simulink model "Hil_Climbers_Integrated_V5"  (R2021a)
settings: Solver=VariableStepAuto  StartTime=0.0  StopTime=10.0  RelTol=1e-3
settings Model: Creator=Sai229  LastModifiedBy=achu

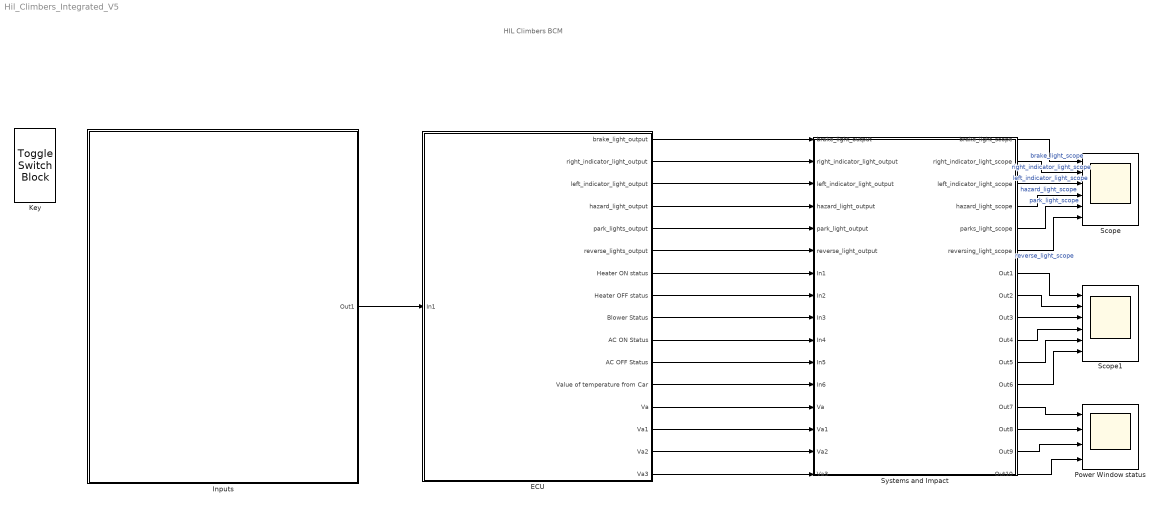
== system Hil_Climbers_Integrated_V5 ==
  note: HIL Climbers BCM
  " ECU" : Subsystem
  Inputs : Subsystem
  Key : ToggleSwitchBlock  LabelPosition=Hide
      settings: Values={{'Off', 'On'}, [0 1]}
  Power Window status : Scope  NumInputPorts=4
  Scope : Scope  NumInputPorts=6
  Scope1 : Scope  NumInputPorts=6
  Systems and Impact : Subsystem
  wires:
  Systems and Impact/12(Out6) -> Scope1/6
  Systems and Impact/11(Out5) -> Scope1/5
  Systems and Impact/10(Out4) -> Scope1/4
  Systems and Impact/1(brake_light_scope) -> Scope/1  "brake_light_scope"
  Systems and Impact/9(Out3) -> Scope1/3
  Systems and Impact/8(Out2) -> Scope1/2
  Systems and Impact/5(parks_light_scope) -> Scope/5  "park_light_scope"
  Systems and Impact/7(Out1) -> Scope1/1
  Systems and Impact/4(hazard_light_scope) -> Scope/4  "hazard_light_scope"
  Systems and Impact/6(reversing_light_scope) -> Scope/6  "reverse_light_scope"
  Systems and Impact/3(left_indicator_light_scope) -> Scope/3  "left_indicator_light_scope"
  Systems and Impact/2(right_indicator_light_scope) -> Scope/2  "right_indicator_light_scope"
  " ECU"/1(brake_light_output) -> Systems and Impact/1(brake_light_output)
  " ECU"/2(right_indicator_light_output) -> Systems and Impact/2(right_indicator_light_output)
  " ECU"/3(left_indicator_light_output) -> Systems and Impact/3(left_indicator_light_output)
  " ECU"/4(hazard_light_output) -> Systems and Impact/4(hazard_light_output)
  " ECU"/5(park_lights_output) -> Systems and Impact/5(park_light_output)
  " ECU"/6(reverse_lights_output) -> Systems and Impact/6(reverse_light_output)
  " ECU"/7(Heater ON status) -> Systems and Impact/7(In1)
  " ECU"/8(Heater OFF status) -> Systems and Impact/8(In2)
  " ECU"/9(Blower Status) -> Systems and Impact/9(In3)
  " ECU"/10(AC ON Status) -> Systems and Impact/10(In4)
  " ECU"/11(AC OFF Status) -> Systems and Impact/11(In5)
  " ECU"/12(Value of temperature from Car) -> Systems and Impact/12(In6)
  " ECU"/13(Va) -> Systems and Impact/13(Va)
  " ECU"/14(Va1) -> Systems and Impact/14(Va1)
  " ECU"/15(Va2) -> Systems and Impact/15(Va2)
  " ECU"/16(Va3) -> Systems and Impact/16(Va3)
  Systems and Impact/13(Out7) -> Power Window status/1
  Systems and Impact/14(Out8) -> Power Window status/2
  Systems and Impact/15(Out9) -> Power Window status/3
  Systems and Impact/16(Out10) -> Power Window status/4
  Inputs/1(Out1) -> " ECU"/1(In1)

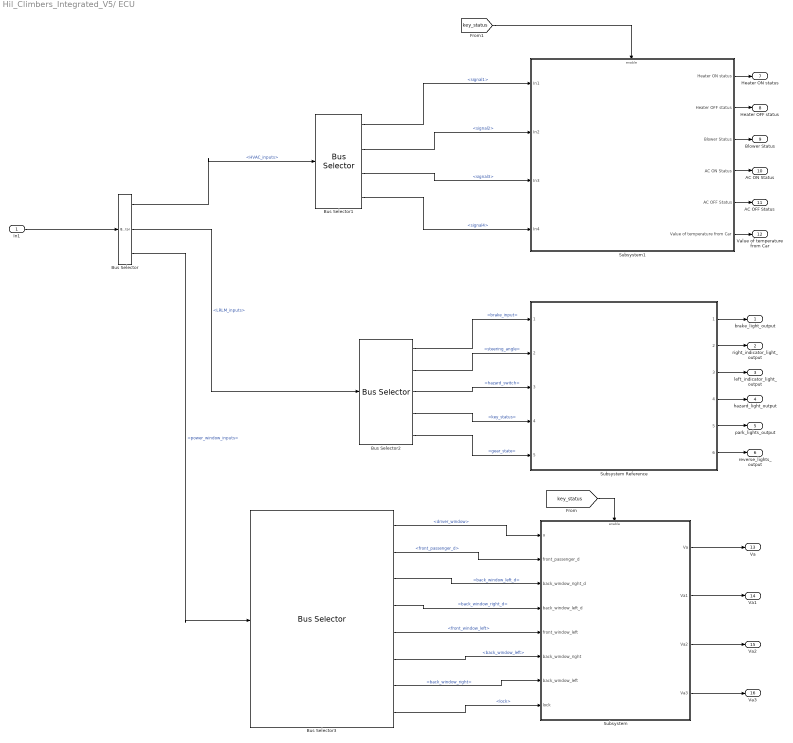
== system Hil_Climbers_Integrated_V5/ ECU ==
  In1 : Inport
  Bus Selector : BusSelector  OutputSignals=HVAC_inputs,LRLM_inputs,power_window_inputs
  Bus Selector1 : BusSelector  OutputSignals=signal1,signal2,signal3,signal4
  Bus Selector2 : BusSelector  OutputSignals=brake_input,steering_angle,hazard_switch,key_status,gear_state
  Bus Selector3 : BusSelector  OutputSignals=driver_window,front_passenger_d,back_window_left_d,back_window_right_d,front_window_left,back_window_left,back_window_right,lock
  Subsystem : Subsystem
  Subsystem Reference : Subsystem  ReferencedSubsystem=LRLM_ECU
  Subsystem1 : Subsystem
  brake_light_output : Outport
  right_indicator_light_output : Outport  Port=2
  left_indicator_light_output : Outport  Port=3
  hazard_light_output : Outport  Port=4
  park_lights_output : Outport  Port=5
  reverse_lights_output : Outport  Port=6
  Heater ON status : Outport  Port=7
  Heater OFF status : Outport  Port=8
  Blower Status : Outport  Port=9
  AC ON Status : Outport  Port=10
  AC OFF Status : Outport  Port=11
  Value of temperature from Car : Outport  Port=12
  Va : Outport  Port=13
  Va1 : Outport  Port=14
  Va2 : Outport  Port=15
  Va3 : Outport  Port=16
  wires:
  Subsystem Reference/5 -> park_lights_output/1
  Subsystem Reference/3 -> left_indicator_light_output/1
  Subsystem Reference/6 -> reverse_lights_output/1
  Subsystem Reference/1 -> brake_light_output/1
  Subsystem Reference/2 -> right_indicator_light_output/1
  Subsystem Reference/4 -> hazard_light_output/1
  Subsystem/1(Va) -> Va/1
  Subsystem/2(Va1) -> Va1/1
  Subsystem/3(Va2) -> Va2/1
  Subsystem/4(Va3) -> Va3/1
  Subsystem1/1(Heater ON status) -> Heater ON status/1
  Subsystem1/2(Heater OFF status) -> Heater OFF status/1
  Subsystem1/3(Blower Status) -> Blower Status/1
  Subsystem1/4(AC ON Status) -> AC ON Status/1
  Subsystem1/5(AC OFF Status) -> AC OFF Status/1
  Subsystem1/6(Value of temperature from Car) -> Value of temperature from Car/1
  [key_status] -> Subsystem1/Enable
  In1/1 -> Bus Selector/1
  Bus Selector/1 -> Bus Selector1/1  "<HVAC_inputs>"
  Bus Selector/2 -> Bus Selector2/1  "<LRLM_inputs>"
  Bus Selector/3 -> Bus Selector3/1  "<power_window_inputs>"
  Bus Selector1/1 -> Subsystem1/1(In1)  "<signal1>"
  Bus Selector1/2 -> Subsystem1/2(In2)  "<signal2>"
  Bus Selector1/3 -> Subsystem1/3(In3)  "<signal3>"
  Bus Selector1/4 -> Subsystem1/4(In4)  "<signal4>"
  Bus Selector3/1 -> Subsystem/1(u)  "<driver_window>"
  Bus Selector3/2 -> Subsystem/2(front_passenger_d)  "<front_passenger_d>"
  Bus Selector3/3 -> Subsystem/3(back_window_right_d)  "<back_window_left_d>"
  Bus Selector3/4 -> Subsystem/4(back_window_left_d)  "<back_window_right_d>"
  Bus Selector3/5 -> Subsystem/5(front_window_left)  "<front_window_left>"
  Bus Selector3/6 -> Subsystem/6(back_window_right)  "<back_window_left>"
  Bus Selector3/7 -> Subsystem/7(back_window_left)  "<back_window_right>"
  Bus Selector3/8 -> Subsystem/8(lock)  "<lock>"
  Bus Selector2/1 -> Subsystem Reference/1  "<brake_input>"
  Bus Selector2/2 -> Subsystem Reference/2  "<steering_angle>"
  Bus Selector2/3 -> Subsystem Reference/3  "<hazard_switch>"
  Bus Selector2/4 -> Subsystem Reference/4  "<key_status>"
  Bus Selector2/5 -> Subsystem Reference/5  "<gear_state>"
  [key_status] -> Subsystem/Enable

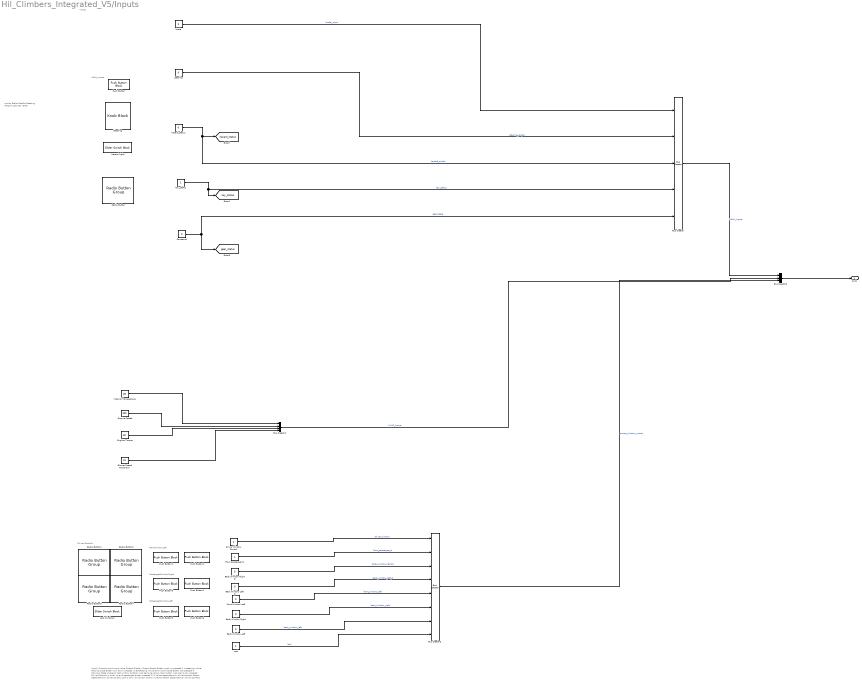
== system Hil_Climbers_Integrated_V5/Inputs ==
  note: Inputs
  note: LRLM_inputs
  note: Inputs:
      | Brake Paddle
      | Steering
      | Hazard Light
      | Key
      | Gear
  note: PsssengertWindowLeft
  note: FrontWindowLeft
  note: Driver Controls
  note: Input / Outputs
      |
      | Input
      | Input value
      | Output Display
      | Output Graph
      |
      | Button push up pressed
      | 1
      | Increasing value
      | Raising slope
      |
      | Button pull down pressed
      | -1
      | Decreasing value
      | Downward slope
      |
      | Button not pressed
      | 0
      | Previous state wherever last window position was
      | Same level as when button was previously pressed
      |
      | Driver Controls in push up and passenger button pressed
      | 1/-1
      | Value dependent on driver controls
      | Graph dependent on driver controls
      |
      | Lock
      | 1
      | Only driver can control windows
      | Graph dependent on driver controls
  note: PsssengertWindowRight
  Back Window Left : Constant  Value=0
  Back Window Left D : Constant  Value=0
  Back Window Right : Constant  Value=0
  Back Window Right D : Constant  Value=0
  Blower Speed Proportion : Constant  Value=10
  Bus Creator : BusCreator  Inputs=5
  Bus Creator1 : BusCreator  Inputs=4
  Bus Creator2 : BusCreator  Inputs=8
  Bus Creator3 : BusCreator  Inputs=3
  Constant4 : Constant  Value=0
  Driver Window Control : Constant
  Engine Speed : Constant  Value=100
  Engine Torque : Constant  Value=30
  Front Window Left : Constant  Value=0
  Front passenger D : Constant
  Hazard Light : SliderSwitchBlock  LabelPosition=Hide
      settings: Values={{'Off', 'On'}, [0 1]}
  Internal Temperature : Constant  Value=28
  Lock : Constant
  Lock Windows : SliderSwitchBlock
      settings: Values={{'Unlock', 'Lock'}, [0 1]}
  Push Button : PushButtonBlock  ButtonText=Brake
  Push Button1 : PushButtonBlock  ButtonText=Push up window
  Push Button2 : PushButtonBlock  ButtonText=Pull down window  OnValue=-1
  Push Button3 : PushButtonBlock  ButtonText=Push up window
  Push Button4 : PushButtonBlock  ButtonText=Pull down window  OnValue=-1
  Push Button5 : PushButtonBlock  ButtonText=Push up window
  Push Button6 : PushButtonBlock  ButtonText=Pull down window  OnValue=-1
  Radio Button : RadioButtonGroup  LabelPosition=Hide  SelectedLabel=Neutral  ButtonGroupName=Gear
      settings: Values={{'Neutral', 'Drive', 'Park', 'Reverse'}, [0 1 2 3]}
  Radio Button1 : RadioButtonGroup  LabelPosition=Hide  SelectedLabel=Open  ButtonGroupName=Driver Window Controls
      settings: Values={{'Open', 'Stop', 'Close'}, [1 0 -1]}
  Radio Button2 : RadioButtonGroup  LabelPosition=Hide  SelectedLabel=Open  ButtonGroupName=Front Passenger
      settings: Values={{'Open', 'Stop', 'Close'}, [1 0 -1]}
  Radio Button3 : RadioButtonGroup  LabelPosition=Hide  SelectedLabel=Stop  ButtonGroupName=Back Window Right
      settings: Values={{'Open', 'Stop', 'Close'}, [1 0 -1]}
  Radio Button4 : RadioButtonGroup  LabelPosition=Hide  SelectedLabel=Stop  ButtonGroupName=Back Window Left
      settings: Values={{'Open', 'Stop', 'Close'}, [1 0 -1]}
  Steering : KnobBlock  LabelPosition=Hide  ScaleMin=-50  ScaleMax=50  TickInterval=10
  brake : Constant  Value=0
  hazard_status : Constant  Value=0
  key_status : Constant
  steering : Constant  Value=0
  Out1 : Outport
  tag scope: gear_status=global, hazard_status=global, key_status=global
  wires:
  brake/1 -> Bus Creator/1  "brake_input"
  Constant4/1 -> Bus Creator/5, [gear_status]  "gear_state"
  steering/1 -> Bus Creator/2  "steering_angle"
  key_status/1 -> Bus Creator/4, [key_status]  "key_status"
  hazard_status/1 -> [hazard_status], Bus Creator/3  "hazard_switch"
  Internal Temperature/1 -> Bus Creator1/1
  Engine Speed/1 -> Bus Creator1/2
  Engine Torque/1 -> Bus Creator1/3
  Blower Speed Proportion/1 -> Bus Creator1/4
  Driver Window Control/1 -> Bus Creator2/1  "driver_window"
  Front passenger D/1 -> Bus Creator2/2  "front_passenger_d"
  Back Window Right D/1 -> Bus Creator2/3  "back_window_right_d"
  Back Window Left D/1 -> Bus Creator2/4  "back_window_left_d"
  Front Window Left/1 -> Bus Creator2/5  "front_window_left"
  Back Window Right/1 -> Bus Creator2/6  "back_window_right"
  Back Window Left/1 -> Bus Creator2/7  "back_window_left"
  Lock/1 -> Bus Creator2/8  "lock"
  Bus Creator/1 -> Bus Creator3/1  "LRLM_inputs"
  Bus Creator1/1 -> Bus Creator3/2  "HVAC_inputs"
  Bus Creator2/1 -> Bus Creator3/3  "power_window_inputs"
  Bus Creator3/1 -> Out1/1

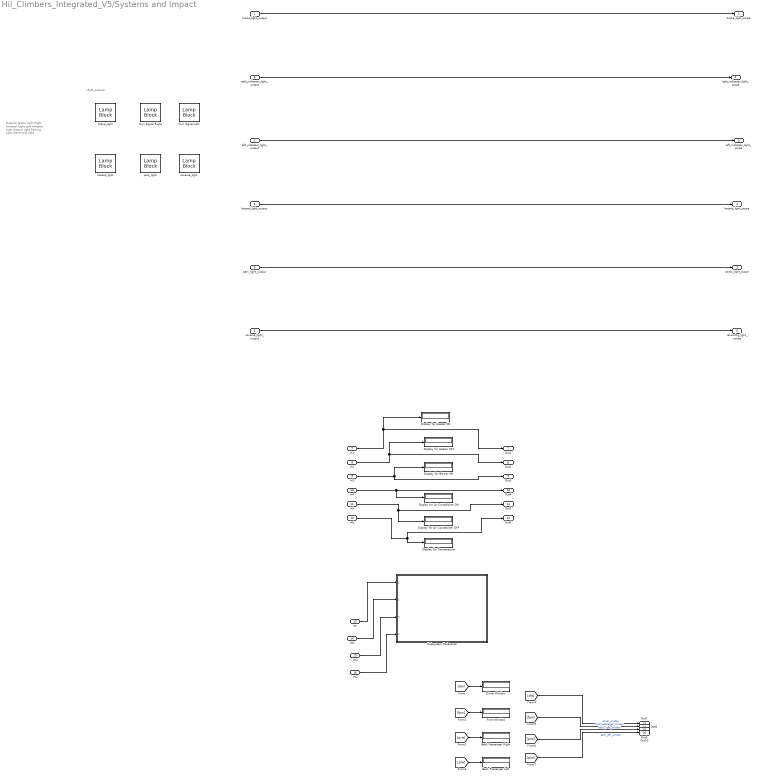
== system Hil_Climbers_Integrated_V5/Systems and Impact ==
  note: Outputs:
      | Brake Light
      | Right Indicator Light
      | Left Indicator Light
      | Hazard Light
      | Parking Light
      | Reversing Light
  note: LRLM_outputs
  brake_light_output : Inport
  right_indicator_light_output : Inport  Port=2
  left_indicator_light_output : Inport  Port=3
  hazard_light_output : Inport  Port=4
  park_light_output : Inport  Port=5
  reverse_light_output : Inport  Port=6
  In1 : Inport  Port=7
  In2 : Inport  Port=8
  In3 : Inport  Port=9
  In4 : Inport  Port=10
  In5 : Inport  Port=11
  In6 : Inport  Port=12
  Va : Inport  Port=13
  Va1 : Inport  Port=14
  Va2 : Inport  Port=15
  Va3 : Inport  Port=16
  Back Passenger Left : Display
  Back Passenger Right : Display
  Display for Air Conditioner OFF : Display
  Display for Air Conditioner ON : Display
  Display for Blower ON : Display
  Display for Heater OFF : Display
  Display for Heater ON : Display
  Display for Temperature : Display
  Driver Window : Display
  Front Window : Display
  Subsystem Reference : Subsystem  ReferencedSubsystem=power_window_system_impact
  Turn Signal Left : LampBlock  LabelPosition=Hide  Icon=TurnSignalLeft
  Turn Signal Right : LampBlock  LabelPosition=Hide  Icon=TurnSignalRight
  brake_light : LampBlock  LabelPosition=Hide  Icon=LightingSwitch
  hazard_light : LampBlock  LabelPosition=Hide  Icon=Hazards
  park_light : LampBlock  Icon=ParkingAssistance
  reverse_light : LampBlock  Icon=RearFogLight
  brake_light_scope : Outport
  right_indicator_light_scope : Outport  Port=2
  left_indicator_light_scope : Outport  Port=3
  hazard_light_scope : Outport  Port=4
  parks_light_scope : Outport  Port=5
  reversing_light_scope : Outport  Port=6
  Out1 : Outport  Port=7
  Out2 : Outport  Port=8
  Out3 : Outport  Port=9
  Out4 : Outport  Port=10
  Out5 : Outport  Port=11
  Out6 : Outport  Port=12
  Out7 : Outport  Port=13
  Out8 : Outport  Port=14
  Out9 : Outport  Port=15
  Out10 : Outport  Port=16
  wires:
  hazard_light_output/1 -> hazard_light_scope/1
  reverse_light_output/1 -> reversing_light_scope/1
  park_light_output/1 -> parks_light_scope/1
  left_indicator_light_output/1 -> left_indicator_light_scope/1
  right_indicator_light_output/1 -> right_indicator_light_scope/1
  brake_light_output/1 -> brake_light_scope/1
  In2/1 -> Out2/1, Display for Heater OFF/1
  In4/1 -> Out4/1, Display for Air Conditioner ON/1
  In3/1 -> Out3/1, Display for Blower ON/1
  In5/1 -> Out5/1, Display for Air Conditioner OFF/1
  In1/1 -> Out1/1, Display for Heater ON/1
  In6/1 -> Out6/1, Display for Temperature/1
  Va/1 -> Subsystem Reference/1
  Va1/1 -> Subsystem Reference/2
  Va2/1 -> Subsystem Reference/3
  Va3/1 -> Subsystem Reference/4
  [plw] -> Back Passenger Left/1
  [prw] -> Back Passenger Right/1
  [fpw] -> Front Window/1
  [dw] -> Out7/1  "driver_window"
  [fpw] -> Out8/1  "front_passenger_window"
  [dw] -> Driver Window/1
  [prw] -> Out9/1  "back_right_window"
  [plw] -> Out10/1  "back_left_window"

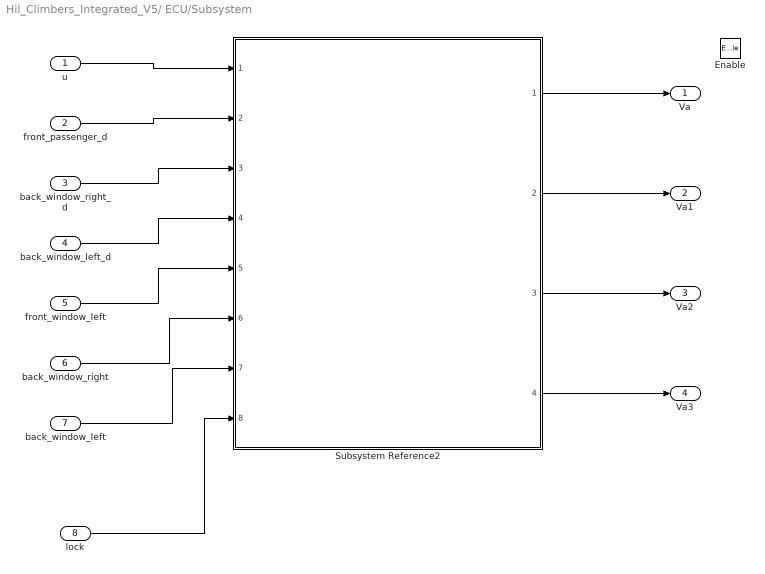
== system Hil_Climbers_Integrated_V5/ ECU/Subsystem ==
  u : Inport
  front_passenger_d : Inport  Port=2
  back_window_right_d : Inport  Port=3
  back_window_left_d : Inport  Port=4
  front_window_left : Inport  Port=5
  back_window_right : Inport  Port=6
  back_window_left : Inport  Port=7
  lock : Inport  Port=8
  Enable : EnablePort  StatesWhenEnabling=reset
  Subsystem Reference2 : Subsystem  ReferencedSubsystem=power_window_ECU
  Va : Outport
  Va1 : Outport  Port=2
  Va2 : Outport  Port=3
  Va3 : Outport  Port=4
  wires:
  Subsystem Reference2/3 -> Va2/1
  Subsystem Reference2/1 -> Va/1
  Subsystem Reference2/2 -> Va1/1
  front_passenger_d/1 -> Subsystem Reference2/2
  back_window_left/1 -> Subsystem Reference2/7
  back_window_right_d/1 -> Subsystem Reference2/3
  back_window_left_d/1 -> Subsystem Reference2/4
  back_window_right/1 -> Subsystem Reference2/6
  Subsystem Reference2/4 -> Va3/1
  front_window_left/1 -> Subsystem Reference2/5
  u/1 -> Subsystem Reference2/1
  lock/1 -> Subsystem Reference2/8

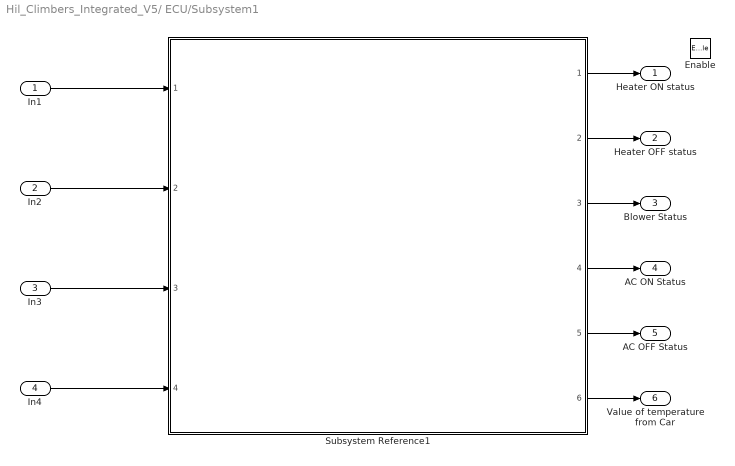
== system Hil_Climbers_Integrated_V5/ ECU/Subsystem1 ==
  In1 : Inport
  In2 : Inport  Port=2
  In3 : Inport  Port=3
  In4 : Inport  Port=4
  Enable : EnablePort  StatesWhenEnabling=reset
  Subsystem Reference1 : Subsystem  ReferencedSubsystem=HVAC_ECU
  Heater ON status : Outport
  Heater OFF status : Outport  Port=2
  Blower Status : Outport  Port=3
  AC ON Status : Outport  Port=4
  AC OFF Status : Outport  Port=5
  Value of temperature from Car : Outport  Port=6
  wires:
  Subsystem Reference1/2 -> Heater OFF status/1
  In2/1 -> Subsystem Reference1/2
  In1/1 -> Subsystem Reference1/1
  Subsystem Reference1/6 -> Value of temperature from Car/1
  Subsystem Reference1/5 -> AC OFF Status/1
  Subsystem Reference1/1 -> Heater ON status/1
  Subsystem Reference1/3 -> Blower Status/1
  In3/1 -> Subsystem Reference1/3
  Subsystem Reference1/4 -> AC ON Status/1
  In4/1 -> Subsystem Reference1/4
